simulink model "TST_HLSDem_SelectParameter"  (R2016b)
settings: Solver=FixedStepDiscrete  StartTime=0.0  StopTime=simTime  FixedStep=sampleTime  RelTol=1e-3
values from neighbouring files (symbols this model uses):
  testCase = 1    [initTST_HLSDem_SelectParameter_001.m]    (also in initTST_HLSDem_SelectParameter_002.m = 2; initTST_HLSDem_SelectParameter_003.m = 3; initTST_HLSDem_SelectParameter_004.m = 4; initTST_HLSDem_SelectParameter_005.m = 5)
libraries: simulink x146, UnitTest_Lib x140
(part 2 of 4)

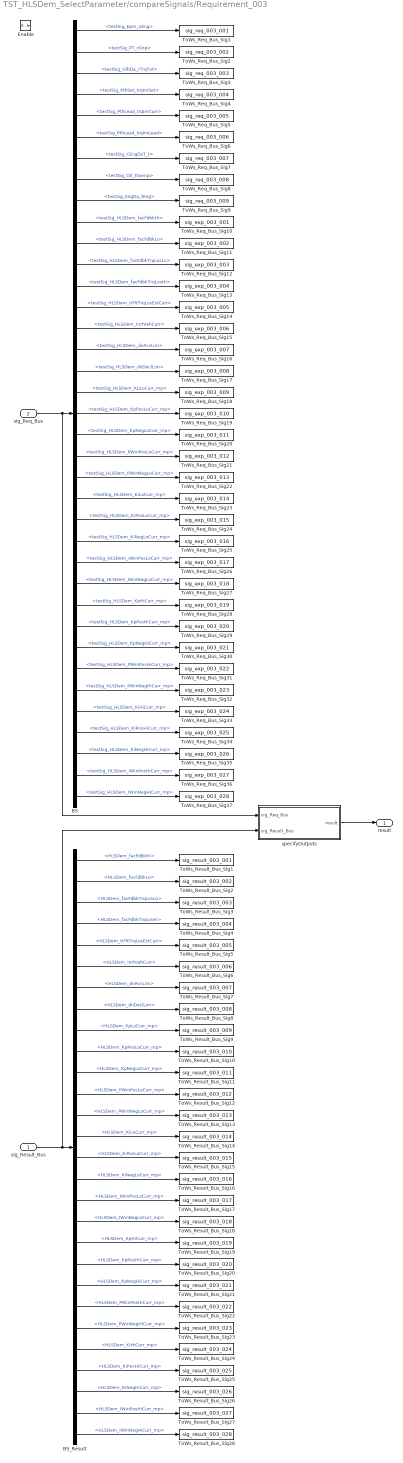
== system TST_HLSDem_SelectParameter/compareSignals/Requirement_003 ==
  sig_Result_Bus : Inport
  sig_Req_Bus : Inport  Port=2
  Enable : EnablePort
  BS : BusSelector  OutputSignals=testSig_Epm_nEng,testSig_PT_rGrip,testSig_GlbDa_rTrqTot,testSig_PthSet_trqInrSet,testSig_PthLead_trqInrCurr,testSig_PthLead_trqInrLead,testSig_CEngDsT_t,testSig_Oil_tSwmp,testSig_EngDa_tEng,testSig_HLSDem_facFdbkHi,testSig_HLSDem_facFdbkLo,testSig_HLSDem_facFdbkTrqLosLo,testSig_HLSDem_facFdbkTrqLosHi,testSig_HLSDem_tiFltTrqLosEstCurr,testSig_HLSDem_InrtVehCurr,testSig_HLSDem_dnAccLim,testSig_HLSDem_dnDeclLim,testSig_HLSDem_KpLoCurr_mp,testSig_HLSDem_KpPosLoCurr_mp,testSig_HLSDem_KpNegLoCurr_mp,testSig_HLSDem_PWinPosLoCurr_mp,testSig_HLSDem_PWinNegLoCurr_mp,testSig_HLSDem_KiLoCurr_mp,testSig_HLSDem_KiPosLoCurr_mp,testSig_HLSDem_KiNegLoCurr_mp,testSig_HLSDem_IWinPosLoCurr_mp,testSig_HLSDem_IWinNegLoCurr_mp,testSig_HLSDem_KpHiCurr_mp,testSig_HLSDem_KpPosHiCurr_mp,testSig_HLSDem_KpNegHiCurr_mp,testSig_HLSDem_PWinPosHiCurr_mp,testSig_HLSDem_PWinNegHiCurr_mp,testSig_HLSDem_KiHiCurr_mp,testSig_HLSDem_KiPosHiCurr_mp,testSig_HLSDem_KiNegHiCurr_mp,testSig_HLSDem_IWinPosHiCurr_mp,testSig_HLSDem_IWinNegHiCurr_mp
  BS_Result : BusSelector  OutputSignals=HLSDem_facFdbkHi,HLSDem_facFdbkLo,HLSDem_facFdbkTrqLosLo,HLSDem_facFdbkTrqLosHi,HLSDem_tiFltTrqLosEstCurr,HLSDem_InrtVehCurr,HLSDem_dnAccLim,HLSDem_dnDeclLim,HLSDem_KpLoCurr_mp,HLSDem_KpPosLoCurr_mp,HLSDem_KpNegLoCurr_mp,HLSDem_PWinPosLoCurr_mp,HLSDem_PWinNegLoCurr_mp,HLSDem_KiLoCurr_mp,HLSDem_KiPosLoCurr_mp,HLSDem_KiNegLoCurr_mp,HLSDem_IWinPosLoCurr_mp,HLSDem_IWinNegLoCurr_mp,HLSDem_KpHiCurr_mp,HLSDem_KpPosHiCurr_mp,HLSDem_KpNegHiCurr_mp,HLSDem_PWinPosHiCurr_mp,HLSDem_PWinNegHiCurr_mp,HLSDem_KiHiCurr_mp,HLSDem_KiPosHiCurr_mp,HLSDem_KiNegHiCurr_mp,HLSDem_IWinPosHiCurr_mp,HLSDem_IWinNegHiCurr_mp
  ToWs_Req_Bus_Sig1 : ToWorkspace  VariableName=sig_req_003_001  SaveFormat=Structure With Time
  ToWs_Req_Bus_Sig10 : ToWorkspace  VariableName=sig_exp_003_001  SaveFormat=Structure With Time
  ToWs_Req_Bus_Sig11 : ToWorkspace  VariableName=sig_exp_003_002  SaveFormat=Structure With Time
  ToWs_Req_Bus_Sig12 : ToWorkspace  VariableName=sig_exp_003_003  SaveFormat=Structure With Time
  ToWs_Req_Bus_Sig13 : ToWorkspace  VariableName=sig_exp_003_004  SaveFormat=Structure With Time
  ToWs_Req_Bus_Sig14 : ToWorkspace  VariableName=sig_exp_003_005  SaveFormat=Structure With Time
  ToWs_Req_Bus_Sig15 : ToWorkspace  VariableName=sig_exp_003_006  SaveFormat=Structure With Time
  ToWs_Req_Bus_Sig16 : ToWorkspace  VariableName=sig_exp_003_007  SaveFormat=Structure With Time
  ToWs_Req_Bus_Sig17 : ToWorkspace  VariableName=sig_exp_003_008  SaveFormat=Structure With Time
  ToWs_Req_Bus_Sig18 : ToWorkspace  VariableName=sig_exp_003_009  SaveFormat=Structure With Time
  ToWs_Req_Bus_Sig19 : ToWorkspace  VariableName=sig_exp_003_010  SaveFormat=Structure With Time
  ToWs_Req_Bus_Sig2 : ToWorkspace  VariableName=sig_req_003_002  SaveFormat=Structure With Time
  ToWs_Req_Bus_Sig20 : ToWorkspace  VariableName=sig_exp_003_011  SaveFormat=Structure With Time
  ToWs_Req_Bus_Sig21 : ToWorkspace  VariableName=sig_exp_003_012  SaveFormat=Structure With Time
  ToWs_Req_Bus_Sig22 : ToWorkspace  VariableName=sig_exp_003_013  SaveFormat=Structure With Time
  ToWs_Req_Bus_Sig23 : ToWorkspace  VariableName=sig_exp_003_014  SaveFormat=Structure With Time
  ToWs_Req_Bus_Sig24 : ToWorkspace  VariableName=sig_exp_003_015  SaveFormat=Structure With Time
  ToWs_Req_Bus_Sig25 : ToWorkspace  VariableName=sig_exp_003_016  SaveFormat=Structure With Time
  ToWs_Req_Bus_Sig26 : ToWorkspace  VariableName=sig_exp_003_017  SaveFormat=Structure With Time
  ToWs_Req_Bus_Sig27 : ToWorkspace  VariableName=sig_exp_003_018  SaveFormat=Structure With Time
  ToWs_Req_Bus_Sig28 : ToWorkspace  VariableName=sig_exp_003_019  SaveFormat=Structure With Time
  ToWs_Req_Bus_Sig29 : ToWorkspace  VariableName=sig_exp_003_020  SaveFormat=Structure With Time
  ToWs_Req_Bus_Sig3 : ToWorkspace  VariableName=sig_req_003_003  SaveFormat=Structure With Time
  ToWs_Req_Bus_Sig30 : ToWorkspace  VariableName=sig_exp_003_021  SaveFormat=Structure With Time
  ToWs_Req_Bus_Sig31 : ToWorkspace  VariableName=sig_exp_003_022  SaveFormat=Structure With Time
  ToWs_Req_Bus_Sig32 : ToWorkspace  VariableName=sig_exp_003_023  SaveFormat=Structure With Time
  ToWs_Req_Bus_Sig33 : ToWorkspace  VariableName=sig_exp_003_024  SaveFormat=Structure With Time
  ToWs_Req_Bus_Sig34 : ToWorkspace  VariableName=sig_exp_003_025  SaveFormat=Structure With Time
  ToWs_Req_Bus_Sig35 : ToWorkspace  VariableName=sig_exp_003_026  SaveFormat=Structure With Time
  ToWs_Req_Bus_Sig36 : ToWorkspace  VariableName=sig_exp_003_027  SaveFormat=Structure With Time
  ToWs_Req_Bus_Sig37 : ToWorkspace  VariableName=sig_exp_003_028  SaveFormat=Structure With Time
  ToWs_Req_Bus_Sig4 : ToWorkspace  VariableName=sig_req_003_004  SaveFormat=Structure With Time
  ToWs_Req_Bus_Sig5 : ToWorkspace  VariableName=sig_req_003_005  SaveFormat=Structure With Time
  ToWs_Req_Bus_Sig6 : ToWorkspace  VariableName=sig_req_003_006  SaveFormat=Structure With Time
  ToWs_Req_Bus_Sig7 : ToWorkspace  VariableName=sig_req_003_007  SaveFormat=Structure With Time
  ToWs_Req_Bus_Sig8 : ToWorkspace  VariableName=sig_req_003_008  SaveFormat=Structure With Time
  ToWs_Req_Bus_Sig9 : ToWorkspace  VariableName=sig_req_003_009  SaveFormat=Structure With Time
  ToWs_Result_Bus_Sig1 : ToWorkspace  VariableName=sig_result_003_001  SaveFormat=Structure With Time
  ToWs_Result_Bus_Sig10 : ToWorkspace  VariableName=sig_result_003_010  SaveFormat=Structure With Time
  ToWs_Result_Bus_Sig11 : ToWorkspace  VariableName=sig_result_003_011  SaveFormat=Structure With Time
  ToWs_Result_Bus_Sig12 : ToWorkspace  VariableName=sig_result_003_012  SaveFormat=Structure With Time
  ToWs_Result_Bus_Sig13 : ToWorkspace  VariableName=sig_result_003_013  SaveFormat=Structure With Time
  ToWs_Result_Bus_Sig14 : ToWorkspace  VariableName=sig_result_003_014  SaveFormat=Structure With Time
  ToWs_Result_Bus_Sig15 : ToWorkspace  VariableName=sig_result_003_015  SaveFormat=Structure With Time
  ToWs_Result_Bus_Sig16 : ToWorkspace  VariableName=sig_result_003_016  SaveFormat=Structure With Time
  ToWs_Result_Bus_Sig17 : ToWorkspace  VariableName=sig_result_003_017  SaveFormat=Structure With Time
  ToWs_Result_Bus_Sig18 : ToWorkspace  VariableName=sig_result_003_018  SaveFormat=Structure With Time
  ToWs_Result_Bus_Sig19 : ToWorkspace  VariableName=sig_result_003_019  SaveFormat=Structure With Time
  ToWs_Result_Bus_Sig2 : ToWorkspace  VariableName=sig_result_003_002  SaveFormat=Structure With Time
  ToWs_Result_Bus_Sig20 : ToWorkspace  VariableName=sig_result_003_020  SaveFormat=Structure With Time
  ToWs_Result_Bus_Sig21 : ToWorkspace  VariableName=sig_result_003_021  SaveFormat=Structure With Time
  ToWs_Result_Bus_Sig22 : ToWorkspace  VariableName=sig_result_003_022  SaveFormat=Structure With Time
  ToWs_Result_Bus_Sig23 : ToWorkspace  VariableName=sig_result_003_023  SaveFormat=Structure With Time
  ToWs_Result_Bus_Sig24 : ToWorkspace  VariableName=sig_result_003_024  SaveFormat=Structure With Time
  ToWs_Result_Bus_Sig25 : ToWorkspace  VariableName=sig_result_003_025  SaveFormat=Structure With Time
  ToWs_Result_Bus_Sig26 : ToWorkspace  VariableName=sig_result_003_026  SaveFormat=Structure With Time
  ToWs_Result_Bus_Sig27 : ToWorkspace  VariableName=sig_result_003_027  SaveFormat=Structure With Time
  ToWs_Result_Bus_Sig28 : ToWorkspace  VariableName=sig_result_003_028  SaveFormat=Structure With Time
  ToWs_Result_Bus_Sig3 : ToWorkspace  VariableName=sig_result_003_003  SaveFormat=Structure With Time
  ToWs_Result_Bus_Sig4 : ToWorkspace  VariableName=sig_result_003_004  SaveFormat=Structure With Time
  ToWs_Result_Bus_Sig5 : ToWorkspace  VariableName=sig_result_003_005  SaveFormat=Structure With Time
  ToWs_Result_Bus_Sig6 : ToWorkspace  VariableName=sig_result_003_006  SaveFormat=Structure With Time
  ToWs_Result_Bus_Sig7 : ToWorkspace  VariableName=sig_result_003_007  SaveFormat=Structure With Time
  ToWs_Result_Bus_Sig8 : ToWorkspace  VariableName=sig_result_003_008  SaveFormat=Structure With Time
  ToWs_Result_Bus_Sig9 : ToWorkspace  VariableName=sig_result_003_009  SaveFormat=Structure With Time
  specifyOutputs : Subsystem
  result : Outport
  wires:
  sig_Req_Bus/1 -> BS/1, specifyOutputs/1(sig_Req_Bus)
  BS/1 -> ToWs_Req_Bus_Sig1/1  "<testSig_Epm_nEng>"
  BS/2 -> ToWs_Req_Bus_Sig2/1  "<testSig_PT_rGrip>"
  BS/3 -> ToWs_Req_Bus_Sig3/1  "<testSig_GlbDa_rTrqTot>"
  BS/4 -> ToWs_Req_Bus_Sig4/1  "<testSig_PthSet_trqInrSet>"
  BS/5 -> ToWs_Req_Bus_Sig5/1  "<testSig_PthLead_trqInrCurr>"
  BS/6 -> ToWs_Req_Bus_Sig6/1  "<testSig_PthLead_trqInrLead>"
  BS/7 -> ToWs_Req_Bus_Sig7/1  "<testSig_CEngDsT_t>"
  BS/8 -> ToWs_Req_Bus_Sig8/1  "<testSig_Oil_tSwmp>"
  BS/9 -> ToWs_Req_Bus_Sig9/1  "<testSig_EngDa_tEng>"
  BS/10 -> ToWs_Req_Bus_Sig10/1  "<testSig_HLSDem_facFdbkHi>"
  BS/11 -> ToWs_Req_Bus_Sig11/1  "<testSig_HLSDem_facFdbkLo>"
  BS/12 -> ToWs_Req_Bus_Sig12/1  "<testSig_HLSDem_facFdbkTrqLosLo>"
  BS/13 -> ToWs_Req_Bus_Sig13/1  "<testSig_HLSDem_facFdbkTrqLosHi>"
  BS/14 -> ToWs_Req_Bus_Sig14/1  "<testSig_HLSDem_tiFltTrqLosEstCurr>"
  BS/15 -> ToWs_Req_Bus_Sig15/1  "<testSig_HLSDem_InrtVehCurr>"
  BS/16 -> ToWs_Req_Bus_Sig16/1  "<testSig_HLSDem_dnAccLim>"
  BS/17 -> ToWs_Req_Bus_Sig17/1  "<testSig_HLSDem_dnDeclLim>"
  BS/18 -> ToWs_Req_Bus_Sig18/1  "<testSig_HLSDem_KpLoCurr_mp>"
  BS/19 -> ToWs_Req_Bus_Sig19/1  "<testSig_HLSDem_KpPosLoCurr_mp>"
  BS/20 -> ToWs_Req_Bus_Sig20/1  "<testSig_HLSDem_KpNegLoCurr_mp>"
  BS/21 -> ToWs_Req_Bus_Sig21/1  "<testSig_HLSDem_PWinPosLoCurr_mp>"
  BS/22 -> ToWs_Req_Bus_Sig22/1  "<testSig_HLSDem_PWinNegLoCurr_mp>"
  BS/23 -> ToWs_Req_Bus_Sig23/1  "<testSig_HLSDem_KiLoCurr_mp>"
  BS/24 -> ToWs_Req_Bus_Sig24/1  "<testSig_HLSDem_KiPosLoCurr_mp>"
  BS/25 -> ToWs_Req_Bus_Sig25/1  "<testSig_HLSDem_KiNegLoCurr_mp>"
  BS/26 -> ToWs_Req_Bus_Sig26/1  "<testSig_HLSDem_IWinPosLoCurr_mp>"
  BS/27 -> ToWs_Req_Bus_Sig27/1  "<testSig_HLSDem_IWinNegLoCurr_mp>"
  BS/28 -> ToWs_Req_Bus_Sig28/1  "<testSig_HLSDem_KpHiCurr_mp>"
  BS/29 -> ToWs_Req_Bus_Sig29/1  "<testSig_HLSDem_KpPosHiCurr_mp>"
  BS/30 -> ToWs_Req_Bus_Sig30/1  "<testSig_HLSDem_KpNegHiCurr_mp>"
  BS/31 -> ToWs_Req_Bus_Sig31/1  "<testSig_HLSDem_PWinPosHiCurr_mp>"
  BS/32 -> ToWs_Req_Bus_Sig32/1  "<testSig_HLSDem_PWinNegHiCurr_mp>"
  BS/33 -> ToWs_Req_Bus_Sig33/1  "<testSig_HLSDem_KiHiCurr_mp>"
  BS/34 -> ToWs_Req_Bus_Sig34/1  "<testSig_HLSDem_KiPosHiCurr_mp>"
  BS/35 -> ToWs_Req_Bus_Sig35/1  "<testSig_HLSDem_KiNegHiCurr_mp>"
  BS/36 -> ToWs_Req_Bus_Sig36/1  "<testSig_HLSDem_IWinPosHiCurr_mp>"
  BS/37 -> ToWs_Req_Bus_Sig37/1  "<testSig_HLSDem_IWinNegHiCurr_mp>"
  sig_Result_Bus/1 -> BS_Result/1, specifyOutputs/2(sig_Result_Bus)
  BS_Result/1 -> ToWs_Result_Bus_Sig1/1  "<HLSDem_facFdbkHi>"
  BS_Result/2 -> ToWs_Result_Bus_Sig2/1  "<HLSDem_facFdbkLo>"
  BS_Result/3 -> ToWs_Result_Bus_Sig3/1  "<HLSDem_facFdbkTrqLosLo>"
  BS_Result/4 -> ToWs_Result_Bus_Sig4/1  "<HLSDem_facFdbkTrqLosHi>"
  BS_Result/5 -> ToWs_Result_Bus_Sig5/1  "<HLSDem_tiFltTrqLosEstCurr>"
  BS_Result/6 -> ToWs_Result_Bus_Sig6/1  "<HLSDem_InrtVehCurr>"
  BS_Result/7 -> ToWs_Result_Bus_Sig7/1  "<HLSDem_dnAccLim>"
  BS_Result/8 -> ToWs_Result_Bus_Sig8/1  "<HLSDem_dnDeclLim>"
  BS_Result/9 -> ToWs_Result_Bus_Sig9/1  "<HLSDem_KpLoCurr_mp>"
  BS_Result/10 -> ToWs_Result_Bus_Sig10/1  "<HLSDem_KpPosLoCurr_mp>"
  BS_Result/11 -> ToWs_Result_Bus_Sig11/1  "<HLSDem_KpNegLoCurr_mp>"
  BS_Result/12 -> ToWs_Result_Bus_Sig12/1  "<HLSDem_PWinPosLoCurr_mp>"
  BS_Result/13 -> ToWs_Result_Bus_Sig13/1  "<HLSDem_PWinNegLoCurr_mp>"
  BS_Result/14 -> ToWs_Result_Bus_Sig14/1  "<HLSDem_KiLoCurr_mp>"
  BS_Result/15 -> ToWs_Result_Bus_Sig15/1  "<HLSDem_KiPosLoCurr_mp>"
  BS_Result/16 -> ToWs_Result_Bus_Sig16/1  "<HLSDem_KiNegLoCurr_mp>"
  BS_Result/17 -> ToWs_Result_Bus_Sig17/1  "<HLSDem_IWinPosLoCurr_mp>"
  BS_Result/18 -> ToWs_Result_Bus_Sig18/1  "<HLSDem_IWinNegLoCurr_mp>"
  BS_Result/19 -> ToWs_Result_Bus_Sig19/1  "<HLSDem_KpHiCurr_mp>"
  BS_Result/20 -> ToWs_Result_Bus_Sig20/1  "<HLSDem_KpPosHiCurr_mp>"
  BS_Result/21 -> ToWs_Result_Bus_Sig21/1  "<HLSDem_KpNegHiCurr_mp>"
  BS_Result/22 -> ToWs_Result_Bus_Sig22/1  "<HLSDem_PWinPosHiCurr_mp>"
  BS_Result/23 -> ToWs_Result_Bus_Sig23/1  "<HLSDem_PWinNegHiCurr_mp>"
  BS_Result/24 -> ToWs_Result_Bus_Sig24/1  "<HLSDem_KiHiCurr_mp>"
  BS_Result/25 -> ToWs_Result_Bus_Sig25/1  "<HLSDem_KiPosHiCurr_mp>"
  BS_Result/26 -> ToWs_Result_Bus_Sig26/1  "<HLSDem_KiNegHiCurr_mp>"
  BS_Result/27 -> ToWs_Result_Bus_Sig27/1  "<HLSDem_IWinPosHiCurr_mp>"
  BS_Result/28 -> ToWs_Result_Bus_Sig28/1  "<HLSDem_IWinNegHiCurr_mp>"
  specifyOutputs/1(result) -> result/1

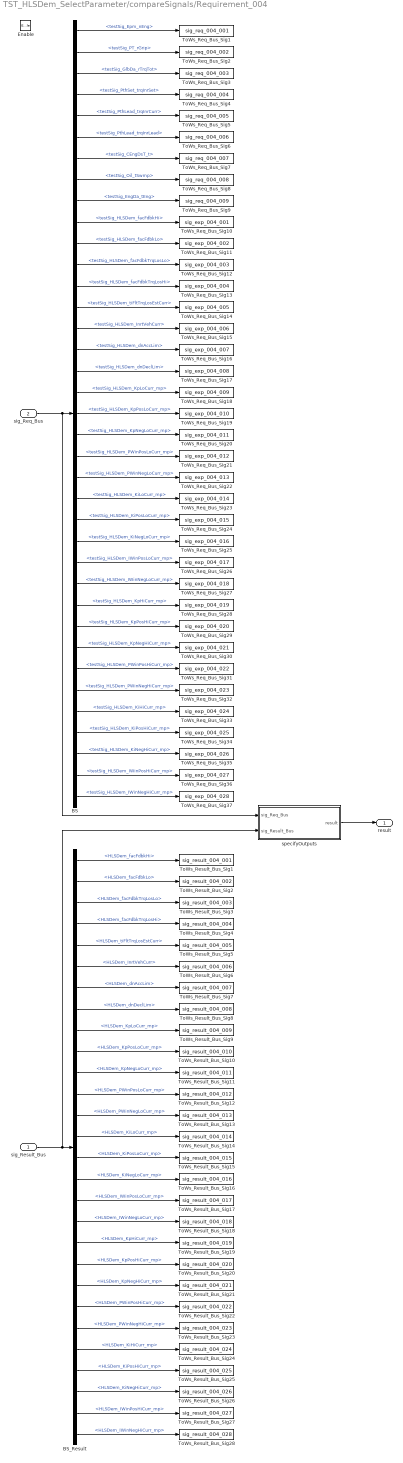
== system TST_HLSDem_SelectParameter/compareSignals/Requirement_004 ==
  sig_Result_Bus : Inport
  sig_Req_Bus : Inport  Port=2
  Enable : EnablePort
  BS : BusSelector  OutputSignals=testSig_Epm_nEng,testSig_PT_rGrip,testSig_GlbDa_rTrqTot,testSig_PthSet_trqInrSet,testSig_PthLead_trqInrCurr,testSig_PthLead_trqInrLead,testSig_CEngDsT_t,testSig_Oil_tSwmp,testSig_EngDa_tEng,testSig_HLSDem_facFdbkHi,testSig_HLSDem_facFdbkLo,testSig_HLSDem_facFdbkTrqLosLo,testSig_HLSDem_facFdbkTrqLosHi,testSig_HLSDem_tiFltTrqLosEstCurr,testSig_HLSDem_InrtVehCurr,testSig_HLSDem_dnAccLim,testSig_HLSDem_dnDeclLim,testSig_HLSDem_KpLoCurr_mp,testSig_HLSDem_KpPosLoCurr_mp,testSig_HLSDem_KpNegLoCurr_mp,testSig_HLSDem_PWinPosLoCurr_mp,testSig_HLSDem_PWinNegLoCurr_mp,testSig_HLSDem_KiLoCurr_mp,testSig_HLSDem_KiPosLoCurr_mp,testSig_HLSDem_KiNegLoCurr_mp,testSig_HLSDem_IWinPosLoCurr_mp,testSig_HLSDem_IWinNegLoCurr_mp,testSig_HLSDem_KpHiCurr_mp,testSig_HLSDem_KpPosHiCurr_mp,testSig_HLSDem_KpNegHiCurr_mp,testSig_HLSDem_PWinPosHiCurr_mp,testSig_HLSDem_PWinNegHiCurr_mp,testSig_HLSDem_KiHiCurr_mp,testSig_HLSDem_KiPosHiCurr_mp,testSig_HLSDem_KiNegHiCurr_mp,testSig_HLSDem_IWinPosHiCurr_mp,testSig_HLSDem_IWinNegHiCurr_mp
  BS_Result : BusSelector  OutputSignals=HLSDem_facFdbkHi,HLSDem_facFdbkLo,HLSDem_facFdbkTrqLosLo,HLSDem_facFdbkTrqLosHi,HLSDem_tiFltTrqLosEstCurr,HLSDem_InrtVehCurr,HLSDem_dnAccLim,HLSDem_dnDeclLim,HLSDem_KpLoCurr_mp,HLSDem_KpPosLoCurr_mp,HLSDem_KpNegLoCurr_mp,HLSDem_PWinPosLoCurr_mp,HLSDem_PWinNegLoCurr_mp,HLSDem_KiLoCurr_mp,HLSDem_KiPosLoCurr_mp,HLSDem_KiNegLoCurr_mp,HLSDem_IWinPosLoCurr_mp,HLSDem_IWinNegLoCurr_mp,HLSDem_KpHiCurr_mp,HLSDem_KpPosHiCurr_mp,HLSDem_KpNegHiCurr_mp,HLSDem_PWinPosHiCurr_mp,HLSDem_PWinNegHiCurr_mp,HLSDem_KiHiCurr_mp,HLSDem_KiPosHiCurr_mp,HLSDem_KiNegHiCurr_mp,HLSDem_IWinPosHiCurr_mp,HLSDem_IWinNegHiCurr_mp
  ToWs_Req_Bus_Sig1 : ToWorkspace  VariableName=sig_req_004_001  SaveFormat=Structure With Time
  ToWs_Req_Bus_Sig10 : ToWorkspace  VariableName=sig_exp_004_001  SaveFormat=Structure With Time
  ToWs_Req_Bus_Sig11 : ToWorkspace  VariableName=sig_exp_004_002  SaveFormat=Structure With Time
  ToWs_Req_Bus_Sig12 : ToWorkspace  VariableName=sig_exp_004_003  SaveFormat=Structure With Time
  ToWs_Req_Bus_Sig13 : ToWorkspace  VariableName=sig_exp_004_004  SaveFormat=Structure With Time
  ToWs_Req_Bus_Sig14 : ToWorkspace  VariableName=sig_exp_004_005  SaveFormat=Structure With Time
  ToWs_Req_Bus_Sig15 : ToWorkspace  VariableName=sig_exp_004_006  SaveFormat=Structure With Time
  ToWs_Req_Bus_Sig16 : ToWorkspace  VariableName=sig_exp_004_007  SaveFormat=Structure With Time
  ToWs_Req_Bus_Sig17 : ToWorkspace  VariableName=sig_exp_004_008  SaveFormat=Structure With Time
  ToWs_Req_Bus_Sig18 : ToWorkspace  VariableName=sig_exp_004_009  SaveFormat=Structure With Time
  ToWs_Req_Bus_Sig19 : ToWorkspace  VariableName=sig_exp_004_010  SaveFormat=Structure With Time
  ToWs_Req_Bus_Sig2 : ToWorkspace  VariableName=sig_req_004_002  SaveFormat=Structure With Time
  ToWs_Req_Bus_Sig20 : ToWorkspace  VariableName=sig_exp_004_011  SaveFormat=Structure With Time
  ToWs_Req_Bus_Sig21 : ToWorkspace  VariableName=sig_exp_004_012  SaveFormat=Structure With Time
  ToWs_Req_Bus_Sig22 : ToWorkspace  VariableName=sig_exp_004_013  SaveFormat=Structure With Time
  ToWs_Req_Bus_Sig23 : ToWorkspace  VariableName=sig_exp_004_014  SaveFormat=Structure With Time
  ToWs_Req_Bus_Sig24 : ToWorkspace  VariableName=sig_exp_004_015  SaveFormat=Structure With Time
  ToWs_Req_Bus_Sig25 : ToWorkspace  VariableName=sig_exp_004_016  SaveFormat=Structure With Time
  ToWs_Req_Bus_Sig26 : ToWorkspace  VariableName=sig_exp_004_017  SaveFormat=Structure With Time
  ToWs_Req_Bus_Sig27 : ToWorkspace  VariableName=sig_exp_004_018  SaveFormat=Structure With Time
  ToWs_Req_Bus_Sig28 : ToWorkspace  VariableName=sig_exp_004_019  SaveFormat=Structure With Time
  ToWs_Req_Bus_Sig29 : ToWorkspace  VariableName=sig_exp_004_020  SaveFormat=Structure With Time
  ToWs_Req_Bus_Sig3 : ToWorkspace  VariableName=sig_req_004_003  SaveFormat=Structure With Time
  ToWs_Req_Bus_Sig30 : ToWorkspace  VariableName=sig_exp_004_021  SaveFormat=Structure With Time
  ToWs_Req_Bus_Sig31 : ToWorkspace  VariableName=sig_exp_004_022  SaveFormat=Structure With Time
  ToWs_Req_Bus_Sig32 : ToWorkspace  VariableName=sig_exp_004_023  SaveFormat=Structure With Time
  ToWs_Req_Bus_Sig33 : ToWorkspace  VariableName=sig_exp_004_024  SaveFormat=Structure With Time
  ToWs_Req_Bus_Sig34 : ToWorkspace  VariableName=sig_exp_004_025  SaveFormat=Structure With Time
  ToWs_Req_Bus_Sig35 : ToWorkspace  VariableName=sig_exp_004_026  SaveFormat=Structure With Time
  ToWs_Req_Bus_Sig36 : ToWorkspace  VariableName=sig_exp_004_027  SaveFormat=Structure With Time
  ToWs_Req_Bus_Sig37 : ToWorkspace  VariableName=sig_exp_004_028  SaveFormat=Structure With Time
  ToWs_Req_Bus_Sig4 : ToWorkspace  VariableName=sig_req_004_004  SaveFormat=Structure With Time
  ToWs_Req_Bus_Sig5 : ToWorkspace  VariableName=sig_req_004_005  SaveFormat=Structure With Time
  ToWs_Req_Bus_Sig6 : ToWorkspace  VariableName=sig_req_004_006  SaveFormat=Structure With Time
  ToWs_Req_Bus_Sig7 : ToWorkspace  VariableName=sig_req_004_007  SaveFormat=Structure With Time
  ToWs_Req_Bus_Sig8 : ToWorkspace  VariableName=sig_req_004_008  SaveFormat=Structure With Time
  ToWs_Req_Bus_Sig9 : ToWorkspace  VariableName=sig_req_004_009  SaveFormat=Structure With Time
  ToWs_Result_Bus_Sig1 : ToWorkspace  VariableName=sig_result_004_001  SaveFormat=Structure With Time
  ToWs_Result_Bus_Sig10 : ToWorkspace  VariableName=sig_result_004_010  SaveFormat=Structure With Time
  ToWs_Result_Bus_Sig11 : ToWorkspace  VariableName=sig_result_004_011  SaveFormat=Structure With Time
  ToWs_Result_Bus_Sig12 : ToWorkspace  VariableName=sig_result_004_012  SaveFormat=Structure With Time
  ToWs_Result_Bus_Sig13 : ToWorkspace  VariableName=sig_result_004_013  SaveFormat=Structure With Time
  ToWs_Result_Bus_Sig14 : ToWorkspace  VariableName=sig_result_004_014  SaveFormat=Structure With Time
  ToWs_Result_Bus_Sig15 : ToWorkspace  VariableName=sig_result_004_015  SaveFormat=Structure With Time
  ToWs_Result_Bus_Sig16 : ToWorkspace  VariableName=sig_result_004_016  SaveFormat=Structure With Time
  ToWs_Result_Bus_Sig17 : ToWorkspace  VariableName=sig_result_004_017  SaveFormat=Structure With Time
  ToWs_Result_Bus_Sig18 : ToWorkspace  VariableName=sig_result_004_018  SaveFormat=Structure With Time
  ToWs_Result_Bus_Sig19 : ToWorkspace  VariableName=sig_result_004_019  SaveFormat=Structure With Time
  ToWs_Result_Bus_Sig2 : ToWorkspace  VariableName=sig_result_004_002  SaveFormat=Structure With Time
  ToWs_Result_Bus_Sig20 : ToWorkspace  VariableName=sig_result_004_020  SaveFormat=Structure With Time
  ToWs_Result_Bus_Sig21 : ToWorkspace  VariableName=sig_result_004_021  SaveFormat=Structure With Time
  ToWs_Result_Bus_Sig22 : ToWorkspace  VariableName=sig_result_004_022  SaveFormat=Structure With Time
  ToWs_Result_Bus_Sig23 : ToWorkspace  VariableName=sig_result_004_023  SaveFormat=Structure With Time
  ToWs_Result_Bus_Sig24 : ToWorkspace  VariableName=sig_result_004_024  SaveFormat=Structure With Time
  ToWs_Result_Bus_Sig25 : ToWorkspace  VariableName=sig_result_004_025  SaveFormat=Structure With Time
  ToWs_Result_Bus_Sig26 : ToWorkspace  VariableName=sig_result_004_026  SaveFormat=Structure With Time
  ToWs_Result_Bus_Sig27 : ToWorkspace  VariableName=sig_result_004_027  SaveFormat=Structure With Time
  ToWs_Result_Bus_Sig28 : ToWorkspace  VariableName=sig_result_004_028  SaveFormat=Structure With Time
  ToWs_Result_Bus_Sig3 : ToWorkspace  VariableName=sig_result_004_003  SaveFormat=Structure With Time
  ToWs_Result_Bus_Sig4 : ToWorkspace  VariableName=sig_result_004_004  SaveFormat=Structure With Time
  ToWs_Result_Bus_Sig5 : ToWorkspace  VariableName=sig_result_004_005  SaveFormat=Structure With Time
  ToWs_Result_Bus_Sig6 : ToWorkspace  VariableName=sig_result_004_006  SaveFormat=Structure With Time
  ToWs_Result_Bus_Sig7 : ToWorkspace  VariableName=sig_result_004_007  SaveFormat=Structure With Time
  ToWs_Result_Bus_Sig8 : ToWorkspace  VariableName=sig_result_004_008  SaveFormat=Structure With Time
  ToWs_Result_Bus_Sig9 : ToWorkspace  VariableName=sig_result_004_009  SaveFormat=Structure With Time
  specifyOutputs : Subsystem
  result : Outport
  wires:
  sig_Req_Bus/1 -> BS/1, specifyOutputs/1(sig_Req_Bus)
  BS/1 -> ToWs_Req_Bus_Sig1/1  "<testSig_Epm_nEng>"
  BS/2 -> ToWs_Req_Bus_Sig2/1  "<testSig_PT_rGrip>"
  BS/3 -> ToWs_Req_Bus_Sig3/1  "<testSig_GlbDa_rTrqTot>"
  BS/4 -> ToWs_Req_Bus_Sig4/1  "<testSig_PthSet_trqInrSet>"
  BS/5 -> ToWs_Req_Bus_Sig5/1  "<testSig_PthLead_trqInrCurr>"
  BS/6 -> ToWs_Req_Bus_Sig6/1  "<testSig_PthLead_trqInrLead>"
  BS/7 -> ToWs_Req_Bus_Sig7/1  "<testSig_CEngDsT_t>"
  BS/8 -> ToWs_Req_Bus_Sig8/1  "<testSig_Oil_tSwmp>"
  BS/9 -> ToWs_Req_Bus_Sig9/1  "<testSig_EngDa_tEng>"
  BS/10 -> ToWs_Req_Bus_Sig10/1  "<testSig_HLSDem_facFdbkHi>"
  BS/11 -> ToWs_Req_Bus_Sig11/1  "<testSig_HLSDem_facFdbkLo>"
  BS/12 -> ToWs_Req_Bus_Sig12/1  "<testSig_HLSDem_facFdbkTrqLosLo>"
  BS/13 -> ToWs_Req_Bus_Sig13/1  "<testSig_HLSDem_facFdbkTrqLosHi>"
  BS/14 -> ToWs_Req_Bus_Sig14/1  "<testSig_HLSDem_tiFltTrqLosEstCurr>"
  BS/15 -> ToWs_Req_Bus_Sig15/1  "<testSig_HLSDem_InrtVehCurr>"
  BS/16 -> ToWs_Req_Bus_Sig16/1  "<testSig_HLSDem_dnAccLim>"
  BS/17 -> ToWs_Req_Bus_Sig17/1  "<testSig_HLSDem_dnDeclLim>"
  BS/18 -> ToWs_Req_Bus_Sig18/1  "<testSig_HLSDem_KpLoCurr_mp>"
  BS/19 -> ToWs_Req_Bus_Sig19/1  "<testSig_HLSDem_KpPosLoCurr_mp>"
  BS/20 -> ToWs_Req_Bus_Sig20/1  "<testSig_HLSDem_KpNegLoCurr_mp>"
  BS/21 -> ToWs_Req_Bus_Sig21/1  "<testSig_HLSDem_PWinPosLoCurr_mp>"
  BS/22 -> ToWs_Req_Bus_Sig22/1  "<testSig_HLSDem_PWinNegLoCurr_mp>"
  BS/23 -> ToWs_Req_Bus_Sig23/1  "<testSig_HLSDem_KiLoCurr_mp>"
  BS/24 -> ToWs_Req_Bus_Sig24/1  "<testSig_HLSDem_KiPosLoCurr_mp>"
  BS/25 -> ToWs_Req_Bus_Sig25/1  "<testSig_HLSDem_KiNegLoCurr_mp>"
  BS/26 -> ToWs_Req_Bus_Sig26/1  "<testSig_HLSDem_IWinPosLoCurr_mp>"
  BS/27 -> ToWs_Req_Bus_Sig27/1  "<testSig_HLSDem_IWinNegLoCurr_mp>"
  BS/28 -> ToWs_Req_Bus_Sig28/1  "<testSig_HLSDem_KpHiCurr_mp>"
  BS/29 -> ToWs_Req_Bus_Sig29/1  "<testSig_HLSDem_KpPosHiCurr_mp>"
  BS/30 -> ToWs_Req_Bus_Sig30/1  "<testSig_HLSDem_KpNegHiCurr_mp>"
  BS/31 -> ToWs_Req_Bus_Sig31/1  "<testSig_HLSDem_PWinPosHiCurr_mp>"
  BS/32 -> ToWs_Req_Bus_Sig32/1  "<testSig_HLSDem_PWinNegHiCurr_mp>"
  BS/33 -> ToWs_Req_Bus_Sig33/1  "<testSig_HLSDem_KiHiCurr_mp>"
  BS/34 -> ToWs_Req_Bus_Sig34/1  "<testSig_HLSDem_KiPosHiCurr_mp>"
  BS/35 -> ToWs_Req_Bus_Sig35/1  "<testSig_HLSDem_KiNegHiCurr_mp>"
  BS/36 -> ToWs_Req_Bus_Sig36/1  "<testSig_HLSDem_IWinPosHiCurr_mp>"
  BS/37 -> ToWs_Req_Bus_Sig37/1  "<testSig_HLSDem_IWinNegHiCurr_mp>"
  sig_Result_Bus/1 -> BS_Result/1, specifyOutputs/2(sig_Result_Bus)
  BS_Result/1 -> ToWs_Result_Bus_Sig1/1  "<HLSDem_facFdbkHi>"
  BS_Result/2 -> ToWs_Result_Bus_Sig2/1  "<HLSDem_facFdbkLo>"
  BS_Result/3 -> ToWs_Result_Bus_Sig3/1  "<HLSDem_facFdbkTrqLosLo>"
  BS_Result/4 -> ToWs_Result_Bus_Sig4/1  "<HLSDem_facFdbkTrqLosHi>"
  BS_Result/5 -> ToWs_Result_Bus_Sig5/1  "<HLSDem_tiFltTrqLosEstCurr>"
  BS_Result/6 -> ToWs_Result_Bus_Sig6/1  "<HLSDem_InrtVehCurr>"
  BS_Result/7 -> ToWs_Result_Bus_Sig7/1  "<HLSDem_dnAccLim>"
  BS_Result/8 -> ToWs_Result_Bus_Sig8/1  "<HLSDem_dnDeclLim>"
  BS_Result/9 -> ToWs_Result_Bus_Sig9/1  "<HLSDem_KpLoCurr_mp>"
  BS_Result/10 -> ToWs_Result_Bus_Sig10/1  "<HLSDem_KpPosLoCurr_mp>"
  BS_Result/11 -> ToWs_Result_Bus_Sig11/1  "<HLSDem_KpNegLoCurr_mp>"
  BS_Result/12 -> ToWs_Result_Bus_Sig12/1  "<HLSDem_PWinPosLoCurr_mp>"
  BS_Result/13 -> ToWs_Result_Bus_Sig13/1  "<HLSDem_PWinNegLoCurr_mp>"
  BS_Result/14 -> ToWs_Result_Bus_Sig14/1  "<HLSDem_KiLoCurr_mp>"
  BS_Result/15 -> ToWs_Result_Bus_Sig15/1  "<HLSDem_KiPosLoCurr_mp>"
  BS_Result/16 -> ToWs_Result_Bus_Sig16/1  "<HLSDem_KiNegLoCurr_mp>"
  BS_Result/17 -> ToWs_Result_Bus_Sig17/1  "<HLSDem_IWinPosLoCurr_mp>"
  BS_Result/18 -> ToWs_Result_Bus_Sig18/1  "<HLSDem_IWinNegLoCurr_mp>"
  BS_Result/19 -> ToWs_Result_Bus_Sig19/1  "<HLSDem_KpHiCurr_mp>"
  BS_Result/20 -> ToWs_Result_Bus_Sig20/1  "<HLSDem_KpPosHiCurr_mp>"
  BS_Result/21 -> ToWs_Result_Bus_Sig21/1  "<HLSDem_KpNegHiCurr_mp>"
  BS_Result/22 -> ToWs_Result_Bus_Sig22/1  "<HLSDem_PWinPosHiCurr_mp>"
  BS_Result/23 -> ToWs_Result_Bus_Sig23/1  "<HLSDem_PWinNegHiCurr_mp>"
  BS_Result/24 -> ToWs_Result_Bus_Sig24/1  "<HLSDem_KiHiCurr_mp>"
  BS_Result/25 -> ToWs_Result_Bus_Sig25/1  "<HLSDem_KiPosHiCurr_mp>"
  BS_Result/26 -> ToWs_Result_Bus_Sig26/1  "<HLSDem_KiNegHiCurr_mp>"
  BS_Result/27 -> ToWs_Result_Bus_Sig27/1  "<HLSDem_IWinPosHiCurr_mp>"
  BS_Result/28 -> ToWs_Result_Bus_Sig28/1  "<HLSDem_IWinNegHiCurr_mp>"
  specifyOutputs/1(result) -> result/1

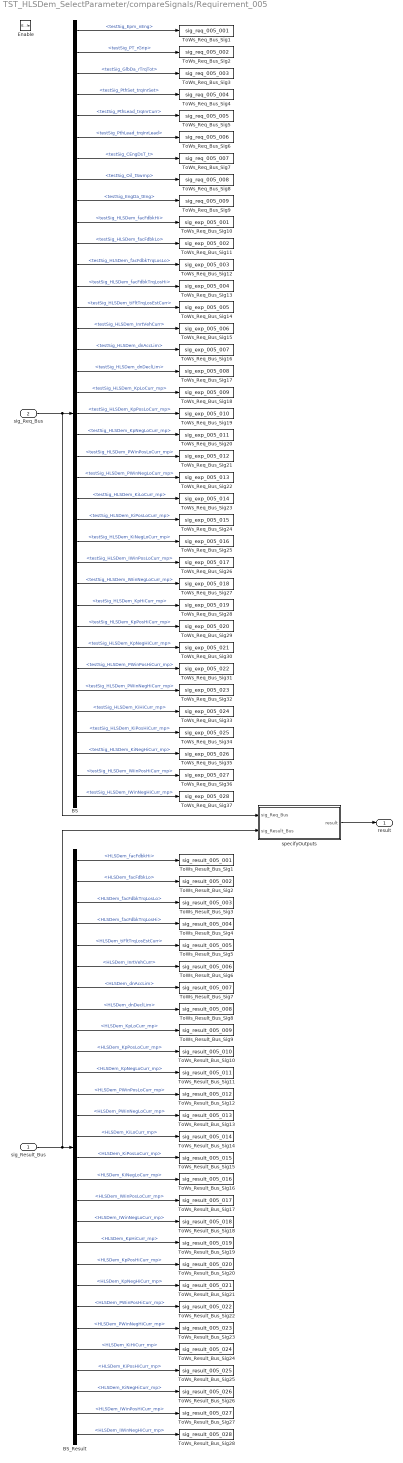
== system TST_HLSDem_SelectParameter/compareSignals/Requirement_005 ==
  sig_Result_Bus : Inport
  sig_Req_Bus : Inport  Port=2
  Enable : EnablePort
  BS : BusSelector  OutputSignals=testSig_Epm_nEng,testSig_PT_rGrip,testSig_GlbDa_rTrqTot,testSig_PthSet_trqInrSet,testSig_PthLead_trqInrCurr,testSig_PthLead_trqInrLead,testSig_CEngDsT_t,testSig_Oil_tSwmp,testSig_EngDa_tEng,testSig_HLSDem_facFdbkHi,testSig_HLSDem_facFdbkLo,testSig_HLSDem_facFdbkTrqLosLo,testSig_HLSDem_facFdbkTrqLosHi,testSig_HLSDem_tiFltTrqLosEstCurr,testSig_HLSDem_InrtVehCurr,testSig_HLSDem_dnAccLim,testSig_HLSDem_dnDeclLim,testSig_HLSDem_KpLoCurr_mp,testSig_HLSDem_KpPosLoCurr_mp,testSig_HLSDem_KpNegLoCurr_mp,testSig_HLSDem_PWinPosLoCurr_mp,testSig_HLSDem_PWinNegLoCurr_mp,testSig_HLSDem_KiLoCurr_mp,testSig_HLSDem_KiPosLoCurr_mp,testSig_HLSDem_KiNegLoCurr_mp,testSig_HLSDem_IWinPosLoCurr_mp,testSig_HLSDem_IWinNegLoCurr_mp,testSig_HLSDem_KpHiCurr_mp,testSig_HLSDem_KpPosHiCurr_mp,testSig_HLSDem_KpNegHiCurr_mp,testSig_HLSDem_PWinPosHiCurr_mp,testSig_HLSDem_PWinNegHiCurr_mp,testSig_HLSDem_KiHiCurr_mp,testSig_HLSDem_KiPosHiCurr_mp,testSig_HLSDem_KiNegHiCurr_mp,testSig_HLSDem_IWinPosHiCurr_mp,testSig_HLSDem_IWinNegHiCurr_mp
  BS_Result : BusSelector  OutputSignals=HLSDem_facFdbkHi,HLSDem_facFdbkLo,HLSDem_facFdbkTrqLosLo,HLSDem_facFdbkTrqLosHi,HLSDem_tiFltTrqLosEstCurr,HLSDem_InrtVehCurr,HLSDem_dnAccLim,HLSDem_dnDeclLim,HLSDem_KpLoCurr_mp,HLSDem_KpPosLoCurr_mp,HLSDem_KpNegLoCurr_mp,HLSDem_PWinPosLoCurr_mp,HLSDem_PWinNegLoCurr_mp,HLSDem_KiLoCurr_mp,HLSDem_KiPosLoCurr_mp,HLSDem_KiNegLoCurr_mp,HLSDem_IWinPosLoCurr_mp,HLSDem_IWinNegLoCurr_mp,HLSDem_KpHiCurr_mp,HLSDem_KpPosHiCurr_mp,HLSDem_KpNegHiCurr_mp,HLSDem_PWinPosHiCurr_mp,HLSDem_PWinNegHiCurr_mp,HLSDem_KiHiCurr_mp,HLSDem_KiPosHiCurr_mp,HLSDem_KiNegHiCurr_mp,HLSDem_IWinPosHiCurr_mp,HLSDem_IWinNegHiCurr_mp
  ToWs_Req_Bus_Sig1 : ToWorkspace  VariableName=sig_req_005_001  SaveFormat=Structure With Time
  ToWs_Req_Bus_Sig10 : ToWorkspace  VariableName=sig_exp_005_001  SaveFormat=Structure With Time
  ToWs_Req_Bus_Sig11 : ToWorkspace  VariableName=sig_exp_005_002  SaveFormat=Structure With Time
  ToWs_Req_Bus_Sig12 : ToWorkspace  VariableName=sig_exp_005_003  SaveFormat=Structure With Time
  ToWs_Req_Bus_Sig13 : ToWorkspace  VariableName=sig_exp_005_004  SaveFormat=Structure With Time
  ToWs_Req_Bus_Sig14 : ToWorkspace  VariableName=sig_exp_005_005  SaveFormat=Structure With Time
  ToWs_Req_Bus_Sig15 : ToWorkspace  VariableName=sig_exp_005_006  SaveFormat=Structure With Time
  ToWs_Req_Bus_Sig16 : ToWorkspace  VariableName=sig_exp_005_007  SaveFormat=Structure With Time
  ToWs_Req_Bus_Sig17 : ToWorkspace  VariableName=sig_exp_005_008  SaveFormat=Structure With Time
  ToWs_Req_Bus_Sig18 : ToWorkspace  VariableName=sig_exp_005_009  SaveFormat=Structure With Time
  ToWs_Req_Bus_Sig19 : ToWorkspace  VariableName=sig_exp_005_010  SaveFormat=Structure With Time
  ToWs_Req_Bus_Sig2 : ToWorkspace  VariableName=sig_req_005_002  SaveFormat=Structure With Time
  ToWs_Req_Bus_Sig20 : ToWorkspace  VariableName=sig_exp_005_011  SaveFormat=Structure With Time
  ToWs_Req_Bus_Sig21 : ToWorkspace  VariableName=sig_exp_005_012  SaveFormat=Structure With Time
  ToWs_Req_Bus_Sig22 : ToWorkspace  VariableName=sig_exp_005_013  SaveFormat=Structure With Time
  ToWs_Req_Bus_Sig23 : ToWorkspace  VariableName=sig_exp_005_014  SaveFormat=Structure With Time
  ToWs_Req_Bus_Sig24 : ToWorkspace  VariableName=sig_exp_005_015  SaveFormat=Structure With Time
  ToWs_Req_Bus_Sig25 : ToWorkspace  VariableName=sig_exp_005_016  SaveFormat=Structure With Time
  ToWs_Req_Bus_Sig26 : ToWorkspace  VariableName=sig_exp_005_017  SaveFormat=Structure With Time
  ToWs_Req_Bus_Sig27 : ToWorkspace  VariableName=sig_exp_005_018  SaveFormat=Structure With Time
  ToWs_Req_Bus_Sig28 : ToWorkspace  VariableName=sig_exp_005_019  SaveFormat=Structure With Time
  ToWs_Req_Bus_Sig29 : ToWorkspace  VariableName=sig_exp_005_020  SaveFormat=Structure With Time
  ToWs_Req_Bus_Sig3 : ToWorkspace  VariableName=sig_req_005_003  SaveFormat=Structure With Time
  ToWs_Req_Bus_Sig30 : ToWorkspace  VariableName=sig_exp_005_021  SaveFormat=Structure With Time
  ToWs_Req_Bus_Sig31 : ToWorkspace  VariableName=sig_exp_005_022  SaveFormat=Structure With Time
  ToWs_Req_Bus_Sig32 : ToWorkspace  VariableName=sig_exp_005_023  SaveFormat=Structure With Time
  ToWs_Req_Bus_Sig33 : ToWorkspace  VariableName=sig_exp_005_024  SaveFormat=Structure With Time
  ToWs_Req_Bus_Sig34 : ToWorkspace  VariableName=sig_exp_005_025  SaveFormat=Structure With Time
  ToWs_Req_Bus_Sig35 : ToWorkspace  VariableName=sig_exp_005_026  SaveFormat=Structure With Time
  ToWs_Req_Bus_Sig36 : ToWorkspace  VariableName=sig_exp_005_027  SaveFormat=Structure With Time
  ToWs_Req_Bus_Sig37 : ToWorkspace  VariableName=sig_exp_005_028  SaveFormat=Structure With Time
  ToWs_Req_Bus_Sig4 : ToWorkspace  VariableName=sig_req_005_004  SaveFormat=Structure With Time
  ToWs_Req_Bus_Sig5 : ToWorkspace  VariableName=sig_req_005_005  SaveFormat=Structure With Time
  ToWs_Req_Bus_Sig6 : ToWorkspace  VariableName=sig_req_005_006  SaveFormat=Structure With Time
  ToWs_Req_Bus_Sig7 : ToWorkspace  VariableName=sig_req_005_007  SaveFormat=Structure With Time
  ToWs_Req_Bus_Sig8 : ToWorkspace  VariableName=sig_req_005_008  SaveFormat=Structure With Time
  ToWs_Req_Bus_Sig9 : ToWorkspace  VariableName=sig_req_005_009  SaveFormat=Structure With Time
  ToWs_Result_Bus_Sig1 : ToWorkspace  VariableName=sig_result_005_001  SaveFormat=Structure With Time
  ToWs_Result_Bus_Sig10 : ToWorkspace  VariableName=sig_result_005_010  SaveFormat=Structure With Time
  ToWs_Result_Bus_Sig11 : ToWorkspace  VariableName=sig_result_005_011  SaveFormat=Structure With Time
  ToWs_Result_Bus_Sig12 : ToWorkspace  VariableName=sig_result_005_012  SaveFormat=Structure With Time
  ToWs_Result_Bus_Sig13 : ToWorkspace  VariableName=sig_result_005_013  SaveFormat=Structure With Time
  ToWs_Result_Bus_Sig14 : ToWorkspace  VariableName=sig_result_005_014  SaveFormat=Structure With Time
  ToWs_Result_Bus_Sig15 : ToWorkspace  VariableName=sig_result_005_015  SaveFormat=Structure With Time
  ToWs_Result_Bus_Sig16 : ToWorkspace  VariableName=sig_result_005_016  SaveFormat=Structure With Time
  ToWs_Result_Bus_Sig17 : ToWorkspace  VariableName=sig_result_005_017  SaveFormat=Structure With Time
  ToWs_Result_Bus_Sig18 : ToWorkspace  VariableName=sig_result_005_018  SaveFormat=Structure With Time
  ToWs_Result_Bus_Sig19 : ToWorkspace  VariableName=sig_result_005_019  SaveFormat=Structure With Time
  ToWs_Result_Bus_Sig2 : ToWorkspace  VariableName=sig_result_005_002  SaveFormat=Structure With Time
  ToWs_Result_Bus_Sig20 : ToWorkspace  VariableName=sig_result_005_020  SaveFormat=Structure With Time
  ToWs_Result_Bus_Sig21 : ToWorkspace  VariableName=sig_result_005_021  SaveFormat=Structure With Time
  ToWs_Result_Bus_Sig22 : ToWorkspace  VariableName=sig_result_005_022  SaveFormat=Structure With Time
  ToWs_Result_Bus_Sig23 : ToWorkspace  VariableName=sig_result_005_023  SaveFormat=Structure With Time
  ToWs_Result_Bus_Sig24 : ToWorkspace  VariableName=sig_result_005_024  SaveFormat=Structure With Time
  ToWs_Result_Bus_Sig25 : ToWorkspace  VariableName=sig_result_005_025  SaveFormat=Structure With Time
  ToWs_Result_Bus_Sig26 : ToWorkspace  VariableName=sig_result_005_026  SaveFormat=Structure With Time
  ToWs_Result_Bus_Sig27 : ToWorkspace  VariableName=sig_result_005_027  SaveFormat=Structure With Time
  ToWs_Result_Bus_Sig28 : ToWorkspace  VariableName=sig_result_005_028  SaveFormat=Structure With Time
  ToWs_Result_Bus_Sig3 : ToWorkspace  VariableName=sig_result_005_003  SaveFormat=Structure With Time
  ToWs_Result_Bus_Sig4 : ToWorkspace  VariableName=sig_result_005_004  SaveFormat=Structure With Time
  ToWs_Result_Bus_Sig5 : ToWorkspace  VariableName=sig_result_005_005  SaveFormat=Structure With Time
  ToWs_Result_Bus_Sig6 : ToWorkspace  VariableName=sig_result_005_006  SaveFormat=Structure With Time
  ToWs_Result_Bus_Sig7 : ToWorkspace  VariableName=sig_result_005_007  SaveFormat=Structure With Time
  ToWs_Result_Bus_Sig8 : ToWorkspace  VariableName=sig_result_005_008  SaveFormat=Structure With Time
  ToWs_Result_Bus_Sig9 : ToWorkspace  VariableName=sig_result_005_009  SaveFormat=Structure With Time
  specifyOutputs : Subsystem
  result : Outport
  wires:
  sig_Req_Bus/1 -> BS/1, specifyOutputs/1(sig_Req_Bus)
  BS/1 -> ToWs_Req_Bus_Sig1/1  "<testSig_Epm_nEng>"
  BS/2 -> ToWs_Req_Bus_Sig2/1  "<testSig_PT_rGrip>"
  BS/3 -> ToWs_Req_Bus_Sig3/1  "<testSig_GlbDa_rTrqTot>"
  BS/4 -> ToWs_Req_Bus_Sig4/1  "<testSig_PthSet_trqInrSet>"
  BS/5 -> ToWs_Req_Bus_Sig5/1  "<testSig_PthLead_trqInrCurr>"
  BS/6 -> ToWs_Req_Bus_Sig6/1  "<testSig_PthLead_trqInrLead>"
  BS/7 -> ToWs_Req_Bus_Sig7/1  "<testSig_CEngDsT_t>"
  BS/8 -> ToWs_Req_Bus_Sig8/1  "<testSig_Oil_tSwmp>"
  BS/9 -> ToWs_Req_Bus_Sig9/1  "<testSig_EngDa_tEng>"
  BS/10 -> ToWs_Req_Bus_Sig10/1  "<testSig_HLSDem_facFdbkHi>"
  BS/11 -> ToWs_Req_Bus_Sig11/1  "<testSig_HLSDem_facFdbkLo>"
  BS/12 -> ToWs_Req_Bus_Sig12/1  "<testSig_HLSDem_facFdbkTrqLosLo>"
  BS/13 -> ToWs_Req_Bus_Sig13/1  "<testSig_HLSDem_facFdbkTrqLosHi>"
  BS/14 -> ToWs_Req_Bus_Sig14/1  "<testSig_HLSDem_tiFltTrqLosEstCurr>"
  BS/15 -> ToWs_Req_Bus_Sig15/1  "<testSig_HLSDem_InrtVehCurr>"
  BS/16 -> ToWs_Req_Bus_Sig16/1  "<testSig_HLSDem_dnAccLim>"
  BS/17 -> ToWs_Req_Bus_Sig17/1  "<testSig_HLSDem_dnDeclLim>"
  BS/18 -> ToWs_Req_Bus_Sig18/1  "<testSig_HLSDem_KpLoCurr_mp>"
  BS/19 -> ToWs_Req_Bus_Sig19/1  "<testSig_HLSDem_KpPosLoCurr_mp>"
  BS/20 -> ToWs_Req_Bus_Sig20/1  "<testSig_HLSDem_KpNegLoCurr_mp>"
  BS/21 -> ToWs_Req_Bus_Sig21/1  "<testSig_HLSDem_PWinPosLoCurr_mp>"
  BS/22 -> ToWs_Req_Bus_Sig22/1  "<testSig_HLSDem_PWinNegLoCurr_mp>"
  BS/23 -> ToWs_Req_Bus_Sig23/1  "<testSig_HLSDem_KiLoCurr_mp>"
  BS/24 -> ToWs_Req_Bus_Sig24/1  "<testSig_HLSDem_KiPosLoCurr_mp>"
  BS/25 -> ToWs_Req_Bus_Sig25/1  "<testSig_HLSDem_KiNegLoCurr_mp>"
  BS/26 -> ToWs_Req_Bus_Sig26/1  "<testSig_HLSDem_IWinPosLoCurr_mp>"
  BS/27 -> ToWs_Req_Bus_Sig27/1  "<testSig_HLSDem_IWinNegLoCurr_mp>"
  BS/28 -> ToWs_Req_Bus_Sig28/1  "<testSig_HLSDem_KpHiCurr_mp>"
  BS/29 -> ToWs_Req_Bus_Sig29/1  "<testSig_HLSDem_KpPosHiCurr_mp>"
  BS/30 -> ToWs_Req_Bus_Sig30/1  "<testSig_HLSDem_KpNegHiCurr_mp>"
  BS/31 -> ToWs_Req_Bus_Sig31/1  "<testSig_HLSDem_PWinPosHiCurr_mp>"
  BS/32 -> ToWs_Req_Bus_Sig32/1  "<testSig_HLSDem_PWinNegHiCurr_mp>"
  BS/33 -> ToWs_Req_Bus_Sig33/1  "<testSig_HLSDem_KiHiCurr_mp>"
  BS/34 -> ToWs_Req_Bus_Sig34/1  "<testSig_HLSDem_KiPosHiCurr_mp>"
  BS/35 -> ToWs_Req_Bus_Sig35/1  "<testSig_HLSDem_KiNegHiCurr_mp>"
  BS/36 -> ToWs_Req_Bus_Sig36/1  "<testSig_HLSDem_IWinPosHiCurr_mp>"
  BS/37 -> ToWs_Req_Bus_Sig37/1  "<testSig_HLSDem_IWinNegHiCurr_mp>"
  sig_Result_Bus/1 -> BS_Result/1, specifyOutputs/2(sig_Result_Bus)
  BS_Result/1 -> ToWs_Result_Bus_Sig1/1  "<HLSDem_facFdbkHi>"
  BS_Result/2 -> ToWs_Result_Bus_Sig2/1  "<HLSDem_facFdbkLo>"
  BS_Result/3 -> ToWs_Result_Bus_Sig3/1  "<HLSDem_facFdbkTrqLosLo>"
  BS_Result/4 -> ToWs_Result_Bus_Sig4/1  "<HLSDem_facFdbkTrqLosHi>"
  BS_Result/5 -> ToWs_Result_Bus_Sig5/1  "<HLSDem_tiFltTrqLosEstCurr>"
  BS_Result/6 -> ToWs_Result_Bus_Sig6/1  "<HLSDem_InrtVehCurr>"
  BS_Result/7 -> ToWs_Result_Bus_Sig7/1  "<HLSDem_dnAccLim>"
  BS_Result/8 -> ToWs_Result_Bus_Sig8/1  "<HLSDem_dnDeclLim>"
  BS_Result/9 -> ToWs_Result_Bus_Sig9/1  "<HLSDem_KpLoCurr_mp>"
  BS_Result/10 -> ToWs_Result_Bus_Sig10/1  "<HLSDem_KpPosLoCurr_mp>"
  BS_Result/11 -> ToWs_Result_Bus_Sig11/1  "<HLSDem_KpNegLoCurr_mp>"
  BS_Result/12 -> ToWs_Result_Bus_Sig12/1  "<HLSDem_PWinPosLoCurr_mp>"
  BS_Result/13 -> ToWs_Result_Bus_Sig13/1  "<HLSDem_PWinNegLoCurr_mp>"
  BS_Result/14 -> ToWs_Result_Bus_Sig14/1  "<HLSDem_KiLoCurr_mp>"
  BS_Result/15 -> ToWs_Result_Bus_Sig15/1  "<HLSDem_KiPosLoCurr_mp>"
  BS_Result/16 -> ToWs_Result_Bus_Sig16/1  "<HLSDem_KiNegLoCurr_mp>"
  BS_Result/17 -> ToWs_Result_Bus_Sig17/1  "<HLSDem_IWinPosLoCurr_mp>"
  BS_Result/18 -> ToWs_Result_Bus_Sig18/1  "<HLSDem_IWinNegLoCurr_mp>"
  BS_Result/19 -> ToWs_Result_Bus_Sig19/1  "<HLSDem_KpHiCurr_mp>"
  BS_Result/20 -> ToWs_Result_Bus_Sig20/1  "<HLSDem_KpPosHiCurr_mp>"
  BS_Result/21 -> ToWs_Result_Bus_Sig21/1  "<HLSDem_KpNegHiCurr_mp>"
  BS_Result/22 -> ToWs_Result_Bus_Sig22/1  "<HLSDem_PWinPosHiCurr_mp>"
  BS_Result/23 -> ToWs_Result_Bus_Sig23/1  "<HLSDem_PWinNegHiCurr_mp>"
  BS_Result/24 -> ToWs_Result_Bus_Sig24/1  "<HLSDem_KiHiCurr_mp>"
  BS_Result/25 -> ToWs_Result_Bus_Sig25/1  "<HLSDem_KiPosHiCurr_mp>"
  BS_Result/26 -> ToWs_Result_Bus_Sig26/1  "<HLSDem_KiNegHiCurr_mp>"
  BS_Result/27 -> ToWs_Result_Bus_Sig27/1  "<HLSDem_IWinPosHiCurr_mp>"
  BS_Result/28 -> ToWs_Result_Bus_Sig28/1  "<HLSDem_IWinNegHiCurr_mp>"
  specifyOutputs/1(result) -> result/1

== system TST_HLSDem_SelectParameter/simulationInput/testSignals_R001 ==
  BC : BusCreator  Inputs=37
  spec_CEngDsT_t : FromWorkspace  VariableName=testSig_CEngDsT_t  Interpolate=off  OutputAfterFinalValue=Holding final value
  spec_EngDa_tEng : FromWorkspace  VariableName=testSig_EngDa_tEng  Interpolate=off  OutputAfterFinalValue=Holding final value
  spec_Epm_nEng : FromWorkspace  VariableName=testSig_Epm_nEng  Interpolate=off  OutputAfterFinalValue=Holding final value
  spec_GlbDa_rTrqTot : FromWorkspace  VariableName=testSig_GlbDa_rTrqTot  Interpolate=off  OutputAfterFinalValue=Holding final value
  spec_HLSDem_IWinNegHiCurr_mp : FromWorkspace  VariableName=testSig_HLSDem_IWinNegHiCurr_mp  Interpolate=off  OutputAfterFinalValue=Holding final value
  spec_HLSDem_IWinNegLoCurr_mp : FromWorkspace  VariableName=testSig_HLSDem_IWinNegLoCurr_mp  Interpolate=off  OutputAfterFinalValue=Holding final value
  spec_HLSDem_IWinPosHiCurr_mp : FromWorkspace  VariableName=testSig_HLSDem_IWinPosHiCurr_mp  Interpolate=off  OutputAfterFinalValue=Holding final value
  spec_HLSDem_IWinPosLoCurr_mp : FromWorkspace  VariableName=testSig_HLSDem_IWinPosLoCurr_mp  Interpolate=off  OutputAfterFinalValue=Holding final value
  spec_HLSDem_InrtVehCurr : FromWorkspace  VariableName=testSig_HLSDem_InrtVehCurr  Interpolate=off  OutputAfterFinalValue=Holding final value
  spec_HLSDem_KiHiCurr_mp : FromWorkspace  VariableName=testSig_HLSDem_KiHiCurr_mp  Interpolate=off  OutputAfterFinalValue=Holding final value
  spec_HLSDem_KiLoCurr_mp : FromWorkspace  VariableName=testSig_HLSDem_KiLoCurr_mp  Interpolate=off  OutputAfterFinalValue=Holding final value
  spec_HLSDem_KiNegHiCurr_mp : FromWorkspace  VariableName=testSig_HLSDem_KiNegHiCurr_mp  Interpolate=off  OutputAfterFinalValue=Holding final value
  spec_HLSDem_KiNegLoCurr_mp : FromWorkspace  VariableName=testSig_HLSDem_KiNegLoCurr_mp  Interpolate=off  OutputAfterFinalValue=Holding final value
  spec_HLSDem_KiPosHiCurr_mp : FromWorkspace  VariableName=testSig_HLSDem_KiPosHiCurr_mp  Interpolate=off  OutputAfterFinalValue=Holding final value
  spec_HLSDem_KiPosLoCurr_mp : FromWorkspace  VariableName=testSig_HLSDem_KiPosLoCurr_mp  Interpolate=off  OutputAfterFinalValue=Holding final value
  spec_HLSDem_KpHiCurr_mp : FromWorkspace  VariableName=testSig_HLSDem_KpHiCurr_mp  Interpolate=off  OutputAfterFinalValue=Holding final value
  spec_HLSDem_KpLoCurr_mp : FromWorkspace  VariableName=testSig_HLSDem_KpLoCurr_mp  Interpolate=off  OutputAfterFinalValue=Holding final value
  spec_HLSDem_KpNegHiCurr_mp : FromWorkspace  VariableName=testSig_HLSDem_KpNegHiCurr_mp  Interpolate=off  OutputAfterFinalValue=Holding final value
  spec_HLSDem_KpNegLoCurr_mp : FromWorkspace  VariableName=testSig_HLSDem_KpNegLoCurr_mp  Interpolate=off  OutputAfterFinalValue=Holding final value
  spec_HLSDem_KpPosHiCurr_mp : FromWorkspace  VariableName=testSig_HLSDem_KpPosHiCurr_mp  Interpolate=off  OutputAfterFinalValue=Holding final value
  spec_HLSDem_KpPosLoCurr_mp : FromWorkspace  VariableName=testSig_HLSDem_KpPosLoCurr_mp  Interpolate=off  OutputAfterFinalValue=Holding final value
  spec_HLSDem_PWinNegHiCurr_mp : FromWorkspace  VariableName=testSig_HLSDem_PWinNegHiCurr_mp  Interpolate=off  OutputAfterFinalValue=Holding final value
  spec_HLSDem_PWinNegLoCurr_mp : FromWorkspace  VariableName=testSig_HLSDem_PWinNegLoCurr_mp  Interpolate=off  OutputAfterFinalValue=Holding final value
  spec_HLSDem_PWinPosHiCurr_mp : FromWorkspace  VariableName=testSig_HLSDem_PWinPosHiCurr_mp  Interpolate=off  OutputAfterFinalValue=Holding final value
  spec_HLSDem_PWinPosLoCurr_mp : FromWorkspace  VariableName=testSig_HLSDem_PWinPosLoCurr_mp  Interpolate=off  OutputAfterFinalValue=Holding final value
  spec_HLSDem_dnAccLim : FromWorkspace  VariableName=testSig_HLSDem_dnAccLim  Interpolate=off  OutputAfterFinalValue=Holding final value
  spec_HLSDem_dnDeclLim : FromWorkspace  VariableName=testSig_HLSDem_dnDeclLim  Interpolate=off  OutputAfterFinalValue=Holding final value
  spec_HLSDem_facFdbkHi : FromWorkspace  VariableName=testSig_HLSDem_facFdbkHi  Interpolate=off  OutputAfterFinalValue=Holding final value
  spec_HLSDem_facFdbkLo : FromWorkspace  VariableName=testSig_HLSDem_facFdbkLo  Interpolate=off  OutputAfterFinalValue=Holding final value
  spec_HLSDem_facFdbkTrqLosHi : FromWorkspace  VariableName=testSig_HLSDem_facFdbkTrqLosHi  Interpolate=off  OutputAfterFinalValue=Holding final value
  spec_HLSDem_facFdbkTrqLosLo : FromWorkspace  VariableName=testSig_HLSDem_facFdbkTrqLosLo  Interpolate=off  OutputAfterFinalValue=Holding final value
  spec_HLSDem_tiFltTrqLosEstCurr : FromWorkspace  VariableName=testSig_HLSDem_tiFltTrqLosEstCurr  Interpolate=off  OutputAfterFinalValue=Holding final value
  spec_Oil_tSwmp : FromWorkspace  VariableName=testSig_Oil_tSwmp  Interpolate=off  OutputAfterFinalValue=Holding final value
  spec_PT_rGrip : FromWorkspace  VariableName=testSig_PT_rGrip  Interpolate=off  OutputAfterFinalValue=Holding final value
  spec_PthLead_trqInrCurr : FromWorkspace  VariableName=testSig_PthLead_trqInrCurr  Interpolate=off  OutputAfterFinalValue=Holding final value
  spec_PthLead_trqInrLead : FromWorkspace  VariableName=testSig_PthLead_trqInrLead  Interpolate=off  OutputAfterFinalValue=Holding final value
  spec_PthSet_trqInrSet : FromWorkspace  VariableName=testSig_PthSet_trqInrSet  Interpolate=off  OutputAfterFinalValue=Holding final value
  testSignals : Outport
  wires:
  BC/1 -> testSignals/1
  spec_Epm_nEng/1 -> BC/1  "testSig_Epm_nEng"
  spec_PT_rGrip/1 -> BC/2  "testSig_PT_rGrip"
  spec_GlbDa_rTrqTot/1 -> BC/3  "testSig_GlbDa_rTrqTot"
  spec_PthSet_trqInrSet/1 -> BC/4  "testSig_PthSet_trqInrSet"
  spec_PthLead_trqInrCurr/1 -> BC/5  "testSig_PthLead_trqInrCurr"
  spec_PthLead_trqInrLead/1 -> BC/6  "testSig_PthLead_trqInrLead"
  spec_CEngDsT_t/1 -> BC/7  "testSig_CEngDsT_t"
  spec_Oil_tSwmp/1 -> BC/8  "testSig_Oil_tSwmp"
  spec_EngDa_tEng/1 -> BC/9  "testSig_EngDa_tEng"
  spec_HLSDem_facFdbkHi/1 -> BC/10  "testSig_HLSDem_facFdbkHi"
  spec_HLSDem_facFdbkLo/1 -> BC/11  "testSig_HLSDem_facFdbkLo"
  spec_HLSDem_facFdbkTrqLosLo/1 -> BC/12  "testSig_HLSDem_facFdbkTrqLosLo"
  spec_HLSDem_facFdbkTrqLosHi/1 -> BC/13  "testSig_HLSDem_facFdbkTrqLosHi"
  spec_HLSDem_tiFltTrqLosEstCurr/1 -> BC/14  "testSig_HLSDem_tiFltTrqLosEstCurr"
  spec_HLSDem_InrtVehCurr/1 -> BC/15  "testSig_HLSDem_InrtVehCurr"
  spec_HLSDem_dnAccLim/1 -> BC/16  "testSig_HLSDem_dnAccLim"
  spec_HLSDem_dnDeclLim/1 -> BC/17  "testSig_HLSDem_dnDeclLim"
  spec_HLSDem_KpLoCurr_mp/1 -> BC/18  "testSig_HLSDem_KpLoCurr_mp"
  spec_HLSDem_KpPosLoCurr_mp/1 -> BC/19  "testSig_HLSDem_KpPosLoCurr_mp"
  spec_HLSDem_KpNegLoCurr_mp/1 -> BC/20  "testSig_HLSDem_KpNegLoCurr_mp"
  spec_HLSDem_PWinPosLoCurr_mp/1 -> BC/21  "testSig_HLSDem_PWinPosLoCurr_mp"
  spec_HLSDem_PWinNegLoCurr_mp/1 -> BC/22  "testSig_HLSDem_PWinNegLoCurr_mp"
  spec_HLSDem_KiLoCurr_mp/1 -> BC/23  "testSig_HLSDem_KiLoCurr_mp"
  spec_HLSDem_KiPosLoCurr_mp/1 -> BC/24  "testSig_HLSDem_KiPosLoCurr_mp"
  spec_HLSDem_KiNegLoCurr_mp/1 -> BC/25  "testSig_HLSDem_KiNegLoCurr_mp"
  spec_HLSDem_IWinPosLoCurr_mp/1 -> BC/26  "testSig_HLSDem_IWinPosLoCurr_mp"
  spec_HLSDem_IWinNegLoCurr_mp/1 -> BC/27  "testSig_HLSDem_IWinNegLoCurr_mp"
  spec_HLSDem_KpHiCurr_mp/1 -> BC/28  "testSig_HLSDem_KpHiCurr_mp"
  spec_HLSDem_KpPosHiCurr_mp/1 -> BC/29  "testSig_HLSDem_KpPosHiCurr_mp"
  spec_HLSDem_KpNegHiCurr_mp/1 -> BC/30  "testSig_HLSDem_KpNegHiCurr_mp"
  spec_HLSDem_PWinPosHiCurr_mp/1 -> BC/31  "testSig_HLSDem_PWinPosHiCurr_mp"
  spec_HLSDem_PWinNegHiCurr_mp/1 -> BC/32  "testSig_HLSDem_PWinNegHiCurr_mp"
  spec_HLSDem_KiHiCurr_mp/1 -> BC/33  "testSig_HLSDem_KiHiCurr_mp"
  spec_HLSDem_KiPosHiCurr_mp/1 -> BC/34  "testSig_HLSDem_KiPosHiCurr_mp"
  spec_HLSDem_KiNegHiCurr_mp/1 -> BC/35  "testSig_HLSDem_KiNegHiCurr_mp"
  spec_HLSDem_IWinPosHiCurr_mp/1 -> BC/36  "testSig_HLSDem_IWinPosHiCurr_mp"
  spec_HLSDem_IWinNegHiCurr_mp/1 -> BC/37  "testSig_HLSDem_IWinNegHiCurr_mp"
